simulink model "gm_biquad_test_v4_old"  (R2024b)
settings: Solver=FixedStepDiscrete  StartTime=0.0  StopTime=T  RelTol=1e-12
undefined symbols (not defined in the file or in its folder): Fs
libraries: dspsrcs4 x1
settings Model: Creator=korvo  LastModifiedBy=korvo
settings OptimizationCC: BlockReduction=off  ConditionallyExecuteInputs=off  DefaultParameterBehavior=Inlined  InheritOutputTypeSmallerThanSingle=on
settings DebuggingCC: AlgebraicLoopMsg=error  ArtificialAlgebraicLoopMsg=error  InheritedTsInSrcMsg=none  SingleTaskRateTransMsg=error  UnconnectedInputMsg=warning  UnconnectedOutputMsg=warning  UnconnectedLineMsg=warning
settings HardwareCC: ProdBitPerPointer=32  ProdBitPerSizeT=32  ProdBitPerPtrDiffT=32  ProdLargestAtomicFloat=None  ProdIntDivRoundTo=Undefined  ProdEndianess=Unspecified  ProdWordSize=32  ProdHWDeviceType=ASIC/FPGA->ASIC/FPGA  TargetBitPerPointer=64  TargetBitPerSizeT=64  TargetBitPerPtrDiffT=64  TargetLongLongMode=on  TargetIntDivRoundTo=Zero  TargetEndianess=LittleEndian  TargetWordSize=64  TargetHWDeviceType=Custom Processor->MATLAB Host Computer  ProdEqTarget=off

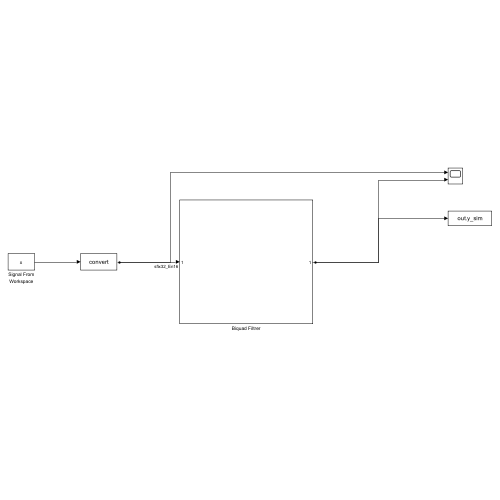
[thumbnail: Simulink's stored preview of the top-level diagram]
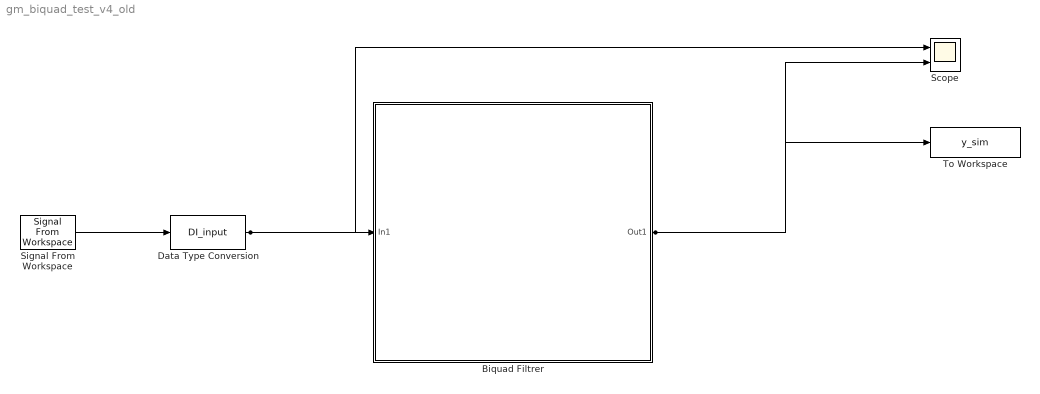
== system gm_biquad_test_v4_old ==
  Biquad Filtrer : Subsystem
  Data Type Conversion : DataTypeConversion  OutDataTypeStr=DI_input  SaturateOnIntegerOverflow=off  RndMeth=Floor
  Scope : Scope  NumInputPorts=2
  Signal From Workspace : dspsrcs4/Signal From Workspace  X=x  Ts=1/Fs  nsamps=1  OutputAfterFinalValue=Setting to zero  ignoreOrWarnInputAndFrameLengths=off  OutputFrames=off
  To Workspace : ToWorkspace  VariableName=y_sim  SampleTime=-1
  wires:
  Biquad Filtrer/1(Out1) -> To Workspace/1, Scope/2
  Data Type Conversion/1 -> Biquad Filtrer/1(In1), Scope/1
  Signal From Workspace/1 -> Data Type Conversion/1

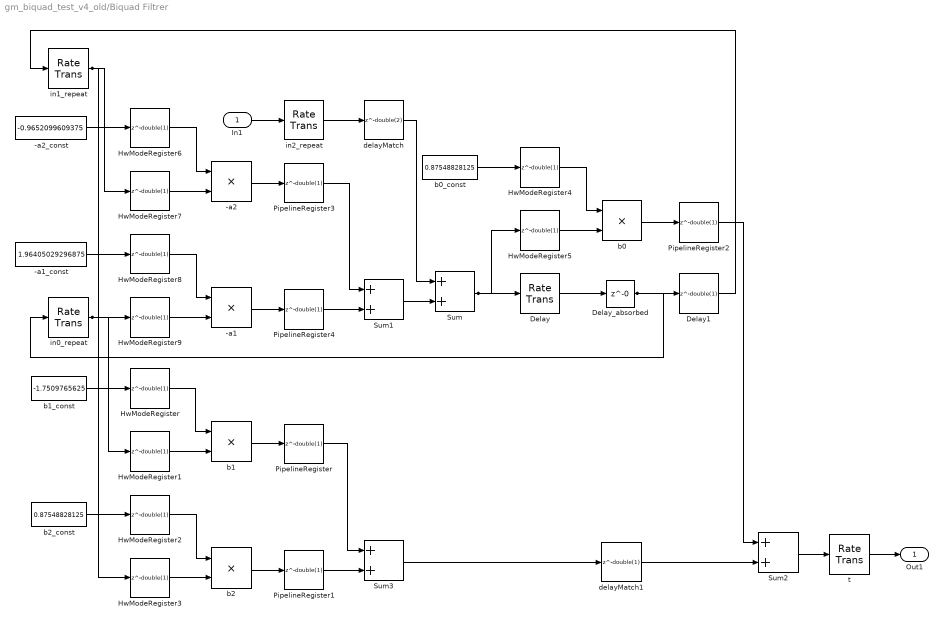
== system gm_biquad_test_v4_old/Biquad Filtrer ==
  In1 : Inport  OutDataTypeStr=fixdt(1, 32, 16)  PortDimensions=1  SampleTime=2.26757369614512e-05
  -a1 : Product  Inputs=**  OutDataTypeStr=fixdt(1, 32, 16)  SampleTime=1.13378684807256e-05
  -a1_const : Constant  Value=1.96405029296875  OutDataTypeStr=fixdt(1, 32, 30)  SampleTime=1.13378684807256e-05
  -a2 : Product  Inputs=**  OutDataTypeStr=fixdt(1, 32, 16)  SampleTime=1.13378684807256e-05
  -a2_const : Constant  Value=-0.9652099609375  OutDataTypeStr=fixdt(1, 32, 31)  SampleTime=1.13378684807256e-05
  Delay : RateTransition  InitialCondition=double(0)  OutPortSampleTimeOpt=Multiple of input port sample time  OutPortSampleTimeMultiple=2
  Delay1 : Delay  DelayLength=double(1)  InitialCondition=0  SampleTime=2.26757369614512e-05
  Delay_absorbed : Delay  DelayLength=0
  HwModeRegister{,1..9} (10 alike) : Delay  DelayLength=double(1)  InitialCondition=0  SampleTime=1.13378684807256e-05
  PipelineRegister{,1..4} (5 alike) : Delay  DelayLength=double(1)  InitialCondition=0  SampleTime=1.13378684807256e-05
  Sum{,1..3} (4 alike) : Sum  OutDataTypeStr=fixdt(1, 32, 16)  AccumDataTypeStr=fixdt(1, 33, 16)  SaturateOnIntegerOverflow=on  SampleTime=1.13378684807256e-05
  b0 : Product  Inputs=**  OutDataTypeStr=fixdt(1, 32, 16)  SampleTime=1.13378684807256e-05
  b0_const : Constant  Value=0.87548828125  OutDataTypeStr=fixdt(1, 32, 31)  SampleTime=1.13378684807256e-05
  b1 : Product  Inputs=**  OutDataTypeStr=fixdt(1, 32, 16)  SampleTime=1.13378684807256e-05
  b1_const : Constant  Value=-1.7509765625  OutDataTypeStr=fixdt(1, 32, 30)  SampleTime=1.13378684807256e-05
  b2 : Product  Inputs=**  OutDataTypeStr=fixdt(1, 32, 16)  SampleTime=1.13378684807256e-05
  b2_const : Constant  Value=0.87548828125  OutDataTypeStr=fixdt(1, 32, 31)  SampleTime=1.13378684807256e-05
  delayMatch : Delay  DelayLength=double(2)  InitialCondition=0  SampleTime=1.13378684807256e-05
  delayMatch1 : Delay  DelayLength=double(1)  InitialCondition=0  SampleTime=1.13378684807256e-05
  in0_repeat : RateTransition  Integrity=off  Deterministic=off  OutPortSampleTimeOpt=Multiple of input port sample time  OutPortSampleTimeMultiple=1/2
  in1_repeat : RateTransition  Integrity=off  Deterministic=off  OutPortSampleTimeOpt=Multiple of input port sample time  OutPortSampleTimeMultiple=1/2
  in2_repeat : RateTransition  Integrity=off  Deterministic=off  OutPortSampleTimeOpt=Multiple of input port sample time  OutPortSampleTimeMultiple=1/2
  t : RateTransition  InitialCondition=double(0)  OutPortSampleTimeOpt=Multiple of input port sample time  OutPortSampleTimeMultiple=2
  Out1 : Outport  SampleTime=2.26757369614512e-05
  wires:
  b1_const/1 -> HwModeRegister/1
  -a1_const/1 -> HwModeRegister8/1
  in1_repeat/1 -> HwModeRegister3/1, HwModeRegister7/1
  b2_const/1 -> HwModeRegister2/1
  in0_repeat/1 -> HwModeRegister1/1, HwModeRegister9/1
  Sum3/1 -> delayMatch1/1
  -a2_const/1 -> HwModeRegister6/1
  HwModeRegister6/1 -> -a2/1
  HwModeRegister7/1 -> -a2/2
  HwModeRegister8/1 -> -a1/1
  HwModeRegister9/1 -> -a1/2
  HwModeRegister/1 -> b1/1
  HwModeRegister1/1 -> b1/2
  HwModeRegister2/1 -> b2/1
  HwModeRegister3/1 -> b2/2
  b2/1 -> PipelineRegister1/1
  In1/1 -> in2_repeat/1
  Sum2/1 -> t/1
  -a2/1 -> PipelineRegister3/1
  -a1/1 -> PipelineRegister4/1
  b1/1 -> PipelineRegister/1
  Delay1/1 -> in1_repeat/1
  in2_repeat/1 -> delayMatch/1
  PipelineRegister3/1 -> Sum1/1
  Delay/1 -> Delay_absorbed/1
  PipelineRegister4/1 -> Sum1/2
  PipelineRegister/1 -> Sum3/1
  PipelineRegister1/1 -> Sum3/2
  delayMatch/1 -> Sum/1
  Sum1/1 -> Sum/2
  b0_const/1 -> HwModeRegister4/1
  Sum/1 -> Delay/1, HwModeRegister5/1
  HwModeRegister4/1 -> b0/1
  HwModeRegister5/1 -> b0/2
  b0/1 -> PipelineRegister2/1
  Delay_absorbed/1 -> Delay1/1, in0_repeat/1
  delayMatch1/1 -> Sum2/2
  PipelineRegister2/1 -> Sum2/1
  t/1 -> Out1/1
